simulink model "Katex_FullCar_R2017b_V03"  (R2026a)
settings: Solver=ode1  StopTime=1000  FixedStep=Ts  EnableMultiTasking=on
PostLoadFcn:
  | , if any(exist('dsrtsu_mdlpostloadfcn', 'file') == [2, 3, 6]), try dsrtsu_mdlpostloadfcn('Execute', bdroot); catch fprintf('Error in PostLoadFcn (dsrtsu_mdlpostloadfcn) for model "%s":\n %s\n', bdroot, lasterr); end, end,
  | , if any(exist('dsrtsu_mdlpostloadfcn', 'file') ~= 0), dsrtsu_mdlpostloadfcn('Execute', bdroot); end,
InitFcn:
  | , if any(exist('rtifpga_mdlclblib', 'file') ~= 0), rtifpga_mdlclblib('Init', bdroot); end,
  | 
  | 
  | init
undefined symbols (not defined in the file): locklim_sus, roundN, Ts
libraries: sl_discontinuities x29, simulink_extras x26, simulink x22, mjLib x1
(part 5 of 10)

== system Katex_FullCar_R2017b_V03/MuJoCo Interface/FR_Motor_Control/Str_Driver/Velocity Mode ==
  In1 : Inport
  Action Port : ActionPort  ActionPortLabel=elseif(u1 == 1)
  Constant : Constant  Value=0
  Terminator : Terminator
  Out1 : Outport  VectorParamsAs1DForOutWhenUnconnected=off
  wires:
  In1/1 -> Terminator/1
  Constant/1 -> Out1/1

== system Katex_FullCar_R2017b_V03/MuJoCo Interface/FR_Motor_Control/Sus_Driver/Position Mode ==
  In1 : Inport
  In2 : Inport  Port=2
  In3 : Inport  Port=3
  In4 : Inport  Port=4
  velocity_rad_s : Inport  Port=5
  Action Port : ActionPort  ActionPortLabel=if(u1 == 0)
  Bus Selector : BusSelector  OutputSignals=FRsus_angref_deg
  Degrees to Radians : simulink_extras/Transformations/Degrees to Radians
  FR_sus_position_motor_driver : Subsystem
  Out1 : Outport  VectorParamsAs1DForOutWhenUnconnected=off
  wires:
  velocity_rad_s/1 -> FR_sus_position_motor_driver/5(velocity_rad_s)
  In4/1 -> FR_sus_position_motor_driver/4(In4)
  In3/1 -> FR_sus_position_motor_driver/3(In3)
  In2/1 -> FR_sus_position_motor_driver/2(In2)
  Bus Selector/1 -> Degrees to Radians/1  "<FRsus_angref_deg>"
  In1/1 -> Bus Selector/1
  FR_sus_position_motor_driver/1(Out1) -> Out1/1
  Degrees to Radians/1 -> FR_sus_position_motor_driver/1(In1)

== system Katex_FullCar_R2017b_V03/MuJoCo Interface/FR_Motor_Control/Sus_Driver/Torque Mode ==
  In1 : Inport
  Action Port : ActionPort  ActionPortLabel=elseif(u1 == 2)
  Bus Selector1 : BusSelector  OutputSignals=FR_tqctrl.FRsus_tqref_pct
  controlgain : Outport  VectorParamsAs1DForOutWhenUnconnected=off
  wires:
  In1/1 -> Bus Selector1/1
  Bus Selector1/1 -> controlgain/1  "<FRsus_tqref_pct>"

== system Katex_FullCar_R2017b_V03/MuJoCo Interface/FR_Motor_Control/Sus_Driver/Velocity Mode ==
  In1 : Inport
  Action Port : ActionPort  ActionPortLabel=elseif(u1 == 1)
  Constant : Constant  Value=0
  Terminator : Terminator
  Out1 : Outport  VectorParamsAs1DForOutWhenUnconnected=off
  wires:
  In1/1 -> Terminator/1
  Constant/1 -> Out1/1

== system Katex_FullCar_R2017b_V03/MuJoCo Interface/RL_Motor_Control/Drv_Driver/Position Mode ==
  In1 : Inport
  Action Port : ActionPort  ActionPortLabel=if(u1 == 0)
  Constant : Constant  Value=0
  Terminator : Terminator
  Out1 : Outport  VectorParamsAs1DForOutWhenUnconnected=off
  wires:
  In1/1 -> Terminator/1
  Constant/1 -> Out1/1

== system Katex_FullCar_R2017b_V03/MuJoCo Interface/RL_Motor_Control/Drv_Driver/Torque Mode ==
  In1 : Inport
  Action Port : ActionPort  ActionPortLabel=elseif(u1 == 2)
  Bus Selector1 : BusSelector  OutputSignals=RL_tqctrl.RLdrv_tqref_pct
  controlgain : Outport  VectorParamsAs1DForOutWhenUnconnected=off
  wires:
  In1/1 -> Bus Selector1/1
  Bus Selector1/1 -> controlgain/1  "<RLdrv_tqref_pct>"

== system Katex_FullCar_R2017b_V03/MuJoCo Interface/RL_Motor_Control/Drv_Driver/Velocity Mode ==
  In1 : Inport
  In2 : Inport  Port=2
  In3 : Inport  Port=3
  In4 : Inport  Port=4
  In5 : Inport  Port=5
  Action Port : ActionPort  ActionPortLabel=elseif(u1 == 1)
  Bus Selector1 : BusSelector  OutputSignals=RLdrv_velref_mps
  RL_vel_velocity_motor_driver : Subsystem
  Subsystem13 : Subsystem
      mask Display: disp('Dri_ref(m/s)_2_motor(rad/s)');
  controlgain : Outport  VectorParamsAs1DForOutWhenUnconnected=off
  wires:
  In5/1 -> Subsystem13/2(In2)
  In4/1 -> RL_vel_velocity_motor_driver/4(In4)
  In3/1 -> RL_vel_velocity_motor_driver/3(In3)
  In2/1 -> RL_vel_velocity_motor_driver/2(In2)
  Subsystem13/1(Out1) -> RL_vel_velocity_motor_driver/1(In1)
  Bus Selector1/1 -> Subsystem13/1(In1)  "<RLdrv_velref_mps>"
  RL_vel_velocity_motor_driver/1(controlgain) -> controlgain/1
  In1/1 -> Bus Selector1/1

== system Katex_FullCar_R2017b_V03/MuJoCo Interface/RL_Motor_Control/Str_Driver/Position Mode ==
  In1 : Inport
  In2 : Inport  Port=2
  In3 : Inport  Port=3
  In4 : Inport  Port=4
  velocity_rad_s : Inport  Port=5
  Action Port : ActionPort  ActionPortLabel=if(u1 == 0)
  Bus Selector1 : BusSelector  OutputSignals=RLstr_angref_deg
  Degrees to Radians1 : simulink_extras/Transformations/Degrees to Radians
  RL_str_position_motor_driver : Subsystem
  Out1 : Outport  VectorParamsAs1DForOutWhenUnconnected=off
  wires:
  velocity_rad_s/1 -> RL_str_position_motor_driver/5(velocity_rad_s)
  In4/1 -> RL_str_position_motor_driver/4(In4)
  In3/1 -> RL_str_position_motor_driver/3(In3)
  In2/1 -> RL_str_position_motor_driver/2(In2)
  RL_str_position_motor_driver/1(Out1) -> Out1/1
  Bus Selector1/1 -> Degrees to Radians1/1  "<RLstr_angref_deg>"
  Degrees to Radians1/1 -> RL_str_position_motor_driver/1(In1)
  In1/1 -> Bus Selector1/1

== system Katex_FullCar_R2017b_V03/MuJoCo Interface/RL_Motor_Control/Str_Driver/Torque Mode ==
  In1 : Inport
  Action Port : ActionPort  ActionPortLabel=elseif(u1 == 2)
  Bus Selector1 : BusSelector  OutputSignals=RL_tqctrl.RLstr_tqref_pct
  controlgain : Outport  VectorParamsAs1DForOutWhenUnconnected=off
  wires:
  Bus Selector1/1 -> controlgain/1  "<RLstr_tqref_pct>"
  In1/1 -> Bus Selector1/1

== system Katex_FullCar_R2017b_V03/MuJoCo Interface/RL_Motor_Control/Str_Driver/Velocity Mode ==
  In1 : Inport
  Action Port : ActionPort  ActionPortLabel=elseif(u1 == 1)
  Constant : Constant  Value=0
  Terminator : Terminator
  Out1 : Outport  VectorParamsAs1DForOutWhenUnconnected=off
  wires:
  In1/1 -> Terminator/1
  Constant/1 -> Out1/1

== system Katex_FullCar_R2017b_V03/MuJoCo Interface/RL_Motor_Control/Sus_Driver/Position Mode ==
  In1 : Inport
  In2 : Inport  Port=2
  In3 : Inport  Port=3
  In4 : Inport  Port=4
  velocity_rad_s : Inport  Port=5
  Action Port : ActionPort  ActionPortLabel=if(u1 == 0)
  Bus Selector : BusSelector  OutputSignals=RLsus_angref_deg
  Degrees to Radians : simulink_extras/Transformations/Degrees to Radians
  RL_sus_position_motor_driver : Subsystem
  Out1 : Outport  VectorParamsAs1DForOutWhenUnconnected=off
  wires:
  velocity_rad_s/1 -> RL_sus_position_motor_driver/5(velocity_rad_s)
  In4/1 -> RL_sus_position_motor_driver/4(In4)
  In3/1 -> RL_sus_position_motor_driver/3(In3)
  In2/1 -> RL_sus_position_motor_driver/2(In2)
  Bus Selector/1 -> Degrees to Radians/1  "<RLsus_angref_deg>"
  In1/1 -> Bus Selector/1
  RL_sus_position_motor_driver/1(Out1) -> Out1/1
  Degrees to Radians/1 -> RL_sus_position_motor_driver/1(In1)

== system Katex_FullCar_R2017b_V03/MuJoCo Interface/RL_Motor_Control/Sus_Driver/Torque Mode ==
  In1 : Inport
  Action Port : ActionPort  ActionPortLabel=elseif(u1 == 2)
  Bus Selector1 : BusSelector  OutputSignals=RL_tqctrl.RLsus_tqref_pct
  controlgain : Outport  VectorParamsAs1DForOutWhenUnconnected=off
  wires:
  In1/1 -> Bus Selector1/1
  Bus Selector1/1 -> controlgain/1  "<RLsus_tqref_pct>"

== system Katex_FullCar_R2017b_V03/MuJoCo Interface/RL_Motor_Control/Sus_Driver/Velocity Mode ==
  In1 : Inport
  Action Port : ActionPort  ActionPortLabel=elseif(u1 == 1)
  Constant : Constant  Value=0
  Terminator : Terminator
  Out1 : Outport  VectorParamsAs1DForOutWhenUnconnected=off
  wires:
  In1/1 -> Terminator/1
  Constant/1 -> Out1/1

== system Katex_FullCar_R2017b_V03/MuJoCo Interface/RR_Motor_Control/Drv_Driver/Position Mode ==
  In1 : Inport
  Action Port : ActionPort  ActionPortLabel=if(u1 == 0)
  Constant : Constant  Value=0
  Terminator : Terminator
  Out1 : Outport  VectorParamsAs1DForOutWhenUnconnected=off
  wires:
  In1/1 -> Terminator/1
  Constant/1 -> Out1/1

== system Katex_FullCar_R2017b_V03/MuJoCo Interface/RR_Motor_Control/Drv_Driver/Torque Mode ==
  In1 : Inport
  Action Port : ActionPort  ActionPortLabel=elseif(u1 == 2)
  Bus Selector1 : BusSelector  OutputSignals=RR_tqctrl.RRdrv_tqref_pct
  controlgain : Outport  VectorParamsAs1DForOutWhenUnconnected=off
  wires:
  In1/1 -> Bus Selector1/1
  Bus Selector1/1 -> controlgain/1  "<RRdrv_tqref_pct>"

== system Katex_FullCar_R2017b_V03/MuJoCo Interface/RR_Motor_Control/Drv_Driver/Velocity Mode ==
  In1 : Inport
  In2 : Inport  Port=2
  In3 : Inport  Port=3
  In4 : Inport  Port=4
  In5 : Inport  Port=5
  Action Port : ActionPort  ActionPortLabel=elseif(u1 == 1)
  Bus Selector1 : BusSelector  OutputSignals=RRdrv_velref_mps
  RR_vel_velocity_motor_driver : Subsystem
  Subsystem13 : Subsystem
      mask Display: disp('Dri_ref(m/s)_2_motor(rad/s)');
  controlgain : Outport  VectorParamsAs1DForOutWhenUnconnected=off
  wires:
  In5/1 -> Subsystem13/2(In2)
  In4/1 -> RR_vel_velocity_motor_driver/4(In4)
  In3/1 -> RR_vel_velocity_motor_driver/3(In3)
  In2/1 -> RR_vel_velocity_motor_driver/2(In2)
  Subsystem13/1(Out1) -> RR_vel_velocity_motor_driver/1(In1)
  Bus Selector1/1 -> Subsystem13/1(In1)  "<RRdrv_velref_mps>"
  RR_vel_velocity_motor_driver/1(controlgain) -> controlgain/1
  In1/1 -> Bus Selector1/1

== system Katex_FullCar_R2017b_V03/MuJoCo Interface/RR_Motor_Control/Str_Driver/Position Mode ==
  In1 : Inport
  In2 : Inport  Port=2
  In3 : Inport  Port=3
  In4 : Inport  Port=4
  velocity_rad_s : Inport  Port=5
  Action Port : ActionPort  ActionPortLabel=if(u1 == 0)
  Bus Selector1 : BusSelector  OutputSignals=RRstr_angref_deg
  Degrees to Radians1 : simulink_extras/Transformations/Degrees to Radians
  RR_str_position_motor_driver : Subsystem
  Out1 : Outport  VectorParamsAs1DForOutWhenUnconnected=off
  wires:
  velocity_rad_s/1 -> RR_str_position_motor_driver/5(velocity_rad_s)
  In4/1 -> RR_str_position_motor_driver/4(In4)
  In3/1 -> RR_str_position_motor_driver/3(In3)
  In2/1 -> RR_str_position_motor_driver/2(In2)
  RR_str_position_motor_driver/1(Out1) -> Out1/1
  Bus Selector1/1 -> Degrees to Radians1/1  "<RRstr_angref_deg>"
  Degrees to Radians1/1 -> RR_str_position_motor_driver/1(In1)
  In1/1 -> Bus Selector1/1

== system Katex_FullCar_R2017b_V03/MuJoCo Interface/RR_Motor_Control/Str_Driver/Torque Mode ==
  In1 : Inport
  Action Port : ActionPort  ActionPortLabel=elseif(u1 == 2)
  Bus Selector1 : BusSelector  OutputSignals=RR_tqctrl.RRstr_tqref_pct
  controlgain : Outport  VectorParamsAs1DForOutWhenUnconnected=off
  wires:
  Bus Selector1/1 -> controlgain/1  "<RRstr_tqref_pct>"
  In1/1 -> Bus Selector1/1

== system Katex_FullCar_R2017b_V03/MuJoCo Interface/RR_Motor_Control/Str_Driver/Velocity Mode ==
  In1 : Inport
  Action Port : ActionPort  ActionPortLabel=elseif(u1 == 1)
  Constant : Constant  Value=0
  Terminator : Terminator
  Out1 : Outport  VectorParamsAs1DForOutWhenUnconnected=off
  wires:
  In1/1 -> Terminator/1
  Constant/1 -> Out1/1

== system Katex_FullCar_R2017b_V03/MuJoCo Interface/RR_Motor_Control/Sus_Driver/Position Mode ==
  In1 : Inport
  In2 : Inport  Port=2
  In3 : Inport  Port=3
  In4 : Inport  Port=4
  velocity_rad_s : Inport  Port=5
  Action Port : ActionPort  ActionPortLabel=if(u1 == 0)
  Bus Selector : BusSelector  OutputSignals=RRsus_angref_deg
  Degrees to Radians : simulink_extras/Transformations/Degrees to Radians
  RR_sus_position_motor_driver : Subsystem
  Out1 : Outport  VectorParamsAs1DForOutWhenUnconnected=off
  wires:
  velocity_rad_s/1 -> RR_sus_position_motor_driver/5(velocity_rad_s)
  In4/1 -> RR_sus_position_motor_driver/4(In4)
  In3/1 -> RR_sus_position_motor_driver/3(In3)
  In2/1 -> RR_sus_position_motor_driver/2(In2)
  Bus Selector/1 -> Degrees to Radians/1  "<RRsus_angref_deg>"
  In1/1 -> Bus Selector/1
  RR_sus_position_motor_driver/1(Out1) -> Out1/1
  Degrees to Radians/1 -> RR_sus_position_motor_driver/1(In1)

== system Katex_FullCar_R2017b_V03/MuJoCo Interface/RR_Motor_Control/Sus_Driver/Torque Mode ==
  In1 : Inport
  Action Port : ActionPort  ActionPortLabel=elseif(u1 == 2)
  Bus Selector1 : BusSelector  OutputSignals=RR_tqctrl.RRsus_tqref_pct
  controlgain : Outport  VectorParamsAs1DForOutWhenUnconnected=off
  wires:
  In1/1 -> Bus Selector1/1
  Bus Selector1/1 -> controlgain/1  "<RRsus_tqref_pct>"

== system Katex_FullCar_R2017b_V03/MuJoCo Interface/RR_Motor_Control/Sus_Driver/Velocity Mode ==
  In1 : Inport
  Action Port : ActionPort  ActionPortLabel=elseif(u1 == 1)
  Constant : Constant  Value=0
  Terminator : Terminator
  Out1 : Outport  VectorParamsAs1DForOutWhenUnconnected=off
  wires:
  In1/1 -> Terminator/1
  Constant/1 -> Out1/1

== system Katex_FullCar_R2017b_V03/DGIST/_High_Level_Ctrl/Chassis_FB_ctrl/Slip contro FLl/Subsystem ==
  Dri_ref[rad/s] : Inport
  Dri_meas[m/s] : Inport  Port=2
  Kgain : Inport  Port=3
  Slip Limit : Inport  Port=4
  radius : Inport  Port=5
  Add : Sum  Inputs=+-
  Constant : Constant  Value=0
  Gain : Gain  Gain=-1
  Max : MinMax  Function=max  Inputs=2
  Min : MinMax  Inputs=2
  "P controller " : Subsystem
  Product : Product
  Product1 : Product
  Product2 : Product
  Saturation Dynamic : sl_discontinuities/Saturation Dynamic  OutMin=[]  OutMax=[]  OutDataTypeStr=Inherit: Same as second input  OutDataType=fixdt(1, 16)  OutScaling=2^-10  DoSatur=off
  Slip_2_omega_block : Subsystem
  Subsystem1 : Subsystem
  re_ref : Scope  NumInputPorts=2
      settings: DataLoggingVariableName=ScopeData3
  ref_meas : Scope  NumInputPorts=2
      settings: DataLoggingVariableName=ScopeData2
  slip ratio : Product  Inputs=*/
  slipratio_satslipratio : Scope  NumInputPorts=2
  omega* : Outport  VectorParamsAs1DForOutWhenUnconnected=off
  wires:
  Dri_meas[m/s]/1 -> ref_meas/2, Slip_2_omega_block/3(Dri_meas[m/s]), Add/2  "Dri_meas[m/s]"
  Kgain/1 -> "P controller "/2(In2)  "Kgain"
  Add/1 -> slip ratio/1, "P controller "/1(In1)  "error[m/s]"
  Slip Limit/1 -> Gain/1, Saturation Dynamic/1  "Slip Limit"
  Gain/1 -> Saturation Dynamic/3
  Saturation Dynamic/1 -> Max/1, slipratio_satslipratio/2, Min/2  "sat slip ratio"
  radius/1 -> Product1/2, Slip_2_omega_block/4(radius)  "radius"
  slip ratio/1 -> slipratio_satslipratio/1  "slip ratio"
  Dri_ref[rad/s]/1 -> [initial_ref], Product1/1  "Dri_ref[rad/s]"
  Product1/1 -> ref_meas/1, Product/2, re_ref/1, slip ratio/2, Add/1  "ref[m/s]"
  Product/1 -> re_ref/2  "re_ref[m/s]"
  Constant/1 -> Min/1, Max/2
  Max/1 -> Slip_2_omega_block/1("lambda+ ")
  Min/1 -> Slip_2_omega_block/2(lambda-)
  Slip_2_omega_block/1(omega*[rad/s]) -> Product/1, omega*/1
  Subsystem1/1(sign) -> Product2/2
  [initial_ref] -> Subsystem1/1(In1)
  "P controller "/1(Out1) -> Product2/1
  Product2/1 -> Saturation Dynamic/2

== system Katex_FullCar_R2017b_V03/DGIST/_High_Level_Ctrl/Chassis_FB_ctrl/Slip control FR/Subsystem ==
  Dri_ref[rad/s] : Inport
  Dri_meas[m/s] : Inport  Port=2
  Kgain : Inport  Port=3
  Slip Limit : Inport  Port=4
  radius : Inport  Port=5
  Add : Sum  Inputs=+-
  Constant : Constant  Value=0
  Gain : Gain  Gain=-1
  Max : MinMax  Function=max  Inputs=2
  Min : MinMax  Inputs=2
  "P controller " : Subsystem
  Product : Product
  Product1 : Product
  Product2 : Product
  Saturation Dynamic : sl_discontinuities/Saturation Dynamic  OutMin=[]  OutMax=[]  OutDataTypeStr=Inherit: Same as second input  OutDataType=fixdt(1, 16)  OutScaling=2^-10  DoSatur=off
  Slip_2_omega_block : Subsystem
  Subsystem1 : Subsystem
  re_ref : Scope  NumInputPorts=2
      settings: DataLoggingVariableName=ScopeData3
  ref_meas : Scope  NumInputPorts=2
      settings: DataLoggingVariableName=ScopeData2
  slip ratio : Product  Inputs=*/
  slipratio_satslipratio : Scope  NumInputPorts=2
  omega* : Outport  VectorParamsAs1DForOutWhenUnconnected=off
  wires:
  Product2/1 -> Saturation Dynamic/2
  "P controller "/1(Out1) -> Product2/1
  [initial_ref] -> Subsystem1/1(In1)
  Subsystem1/1(sign) -> Product2/2
  Slip_2_omega_block/1(omega*[rad/s]) -> omega*/1, Product/1
  Min/1 -> Slip_2_omega_block/2(lambda-)
  Max/1 -> Slip_2_omega_block/1("lambda+ ")
  Constant/1 -> Max/2, Min/1
  Product/1 -> re_ref/2  "re_ref[m/s]"
  Product1/1 -> Add/1, slip ratio/2, re_ref/1, Product/2, ref_meas/1  "ref[m/s]"
  Dri_ref[rad/s]/1 -> Product1/1, [initial_ref]  "Dri_ref[rad/s]"
  slip ratio/1 -> slipratio_satslipratio/1  "slip ratio"
  radius/1 -> Slip_2_omega_block/4(radius), Product1/2  "radius"
  Saturation Dynamic/1 -> Min/2, slipratio_satslipratio/2, Max/1  "sat slip ratio"
  Gain/1 -> Saturation Dynamic/3
  Slip Limit/1 -> Saturation Dynamic/1, Gain/1  "Slip Limit"
  Add/1 -> "P controller "/1(In1), slip ratio/1  "error[m/s]"
  Kgain/1 -> "P controller "/2(In2)  "Kgain"
  Dri_meas[m/s]/1 -> Add/2, Slip_2_omega_block/3(Dri_meas[m/s]), ref_meas/2  "Dri_meas[m/s]"

== system Katex_FullCar_R2017b_V03/DGIST/_High_Level_Ctrl/Chassis_FB_ctrl/Subsystem3/If Action Subsystem ==
  In1 : Inport
  Action Port : ActionPort  ActionPortLabel=if(u1 >= 0)
  Out1 : Outport  VectorParamsAs1DForOutWhenUnconnected=off
  wires:
  In1/1 -> Out1/1

== system Katex_FullCar_R2017b_V03/DGIST/_High_Level_Ctrl/Chassis_FB_ctrl/Subsystem3/If Action Subsystem1 ==
  In1 : Inport
  Action Port : ActionPort  ActionPortLabel=elseif(u1<0)
  Out1 : Outport  VectorParamsAs1DForOutWhenUnconnected=off
  wires:
  In1/1 -> Out1/1

== system Katex_FullCar_R2017b_V03/DGIST/_Low_Level_Ctrl/Driving_Low_Level_Controller/FB Mode/Dri_Loadradps_2_mps ==
  note: Load rad/s
  note: Load m/s
  In1 : Inport
  Product7 : Product
  wheel_radius1 : Constant  Value=0.15
  Out1 : Outport
  wires:
  Product7/1 -> Out1/1
  In1/1 -> Product7/1
  wheel_radius1/1 -> Product7/2

== system Katex_FullCar_R2017b_V03/DGIST/_Low_Level_Ctrl/Driving_Low_Level_Controller/FB Mode/Dri_Loadradps_2_mps1 ==
  note: Load rad/s
  note: Load m/s
  In1 : Inport
  Product7 : Product
  wheel_radius1 : Constant  Value=0.15
  Out1 : Outport
  wires:
  Product7/1 -> Out1/1
  In1/1 -> Product7/1
  wheel_radius1/1 -> Product7/2

== system Katex_FullCar_R2017b_V03/DGIST/_Low_Level_Ctrl/Driving_Low_Level_Controller/Torque Mode/Driving Wheel Control ==
  note: DOB => 이전 Unsaturated Torque를 사용하는게 아니고
      | 이전 실제 Applied/Saturation Torque를 사용 필요?
      | (생각해봐야함)
  note: okay
  note: okay
  note: okay
  Ref : Inport
  Measure : Inport  Port=2
  Add : Sum  Inputs=++-
  Add1 : Sum  Inputs=+-
  Constant : Constant  Value=0
  DOB(omega) : Subsystem
  Feedforward(omega) : Subsystem
  Poleplacement(PI)1 : Subsystem
  Subsystem : Subsystem
  Target Torque : Outport
  tag scope: DriFR_ctrl_FF=global, DriFR_ctrl_PID=global, DriFR_ctrl_Total=global, DriFR_ctrl_dhat=global
  wires:
  Ref/1 -> Add1/1, Feedforward(omega)/1(command)  "Load rad/s"
  [dri_ff_cutoff] -> Feedforward(omega)/2(LFP cutoff)
  Subsystem/1(Target Torque) -> Target Torque/1
  Feedforward(omega)/1(FF) -> [DriFR_ctrl_FF], Add/1
  Poleplacement(PI)1/1(feedback gain) -> [DriFR_ctrl_PID], Add/2
  [Sensor_wheel_angvel] -> DOB(omega)/2(Y_out(w))
  DOB(omega)/1(Dist_hat) -> [DriFR_ctrl_dhat], Add/3
  Add/1 -> DOB(omega)/1(U_in*(Tm)), [DriFR_ctrl_Total], Subsystem/1(N*m)
  [dri_ff_onoff] -> Feedforward(omega)/3(ControlOnOff)
  [dri_dob_onoff] -> DOB(omega)/4(ControlOnOff)
  [dri_dob_cutoff] -> DOB(omega)/3(CutoffFreq_Q)
  [dri_pid_zeta] -> Poleplacement(PI)1/3(zeta)
  Measure/1 -> Add1/2  "Load rad/s"
  Add1/1 -> Poleplacement(PI)1/1(error)
  [dri_pid_cutoff] -> Poleplacement(PI)1/2(BW)
  [dri_pid_onoff] -> Poleplacement(PI)1/4(ConstrolOnOff)
  Constant/1 -> Poleplacement(PI)1/5(ControlInputError)

== system Katex_FullCar_R2017b_V03/DGIST/_Low_Level_Ctrl/Driving_Low_Level_Controller/Velocity Mode/Dri_Loadradps_2_mps ==
  note: Load rad/s
  note: Load m/s
  In1 : Inport
  Product7 : Product
  wheel_radius1 : Constant  Value=0.15
  Out1 : Outport
  wires:
  Product7/1 -> Out1/1
  In1/1 -> Product7/1
  wheel_radius1/1 -> Product7/2

== system Katex_FullCar_R2017b_V03/DGIST/_Low_Level_Ctrl/Driving_Low_Level_Controller/Velocity Mode/Dri_Loadradps_2_mps1 ==
  note: Load rad/s
  note: Load m/s
  In1 : Inport
  Product7 : Product
  wheel_radius1 : Constant  Value=0.15
  Out1 : Outport
  wires:
  Product7/1 -> Out1/1
  In1/1 -> Product7/1
  wheel_radius1/1 -> Product7/2

== system Katex_FullCar_R2017b_V03/DGIST/_Low_Level_Ctrl/Driving_Low_Level_Controller/Velocity Mode/Dri_Loadradps_2_mps2 ==
  note: Load rad/s
  note: Load m/s
  In1 : Inport
  Product7 : Product
  wheel_radius1 : Constant  Value=0.15
  Out1 : Outport
  wires:
  Product7/1 -> Out1/1
  In1/1 -> Product7/1
  wheel_radius1/1 -> Product7/2

== system Katex_FullCar_R2017b_V03/DGIST/_Low_Level_Ctrl/Driving_Low_Level_Controller/Velocity Mode/Dri_Loadradps_2_mps3 ==
  note: Load rad/s
  note: Load m/s
  In1 : Inport
  Product7 : Product
  wheel_radius1 : Constant  Value=0.15
  Out1 : Outport
  wires:
  Product7/1 -> Out1/1
  In1/1 -> Product7/1
  wheel_radius1/1 -> Product7/2

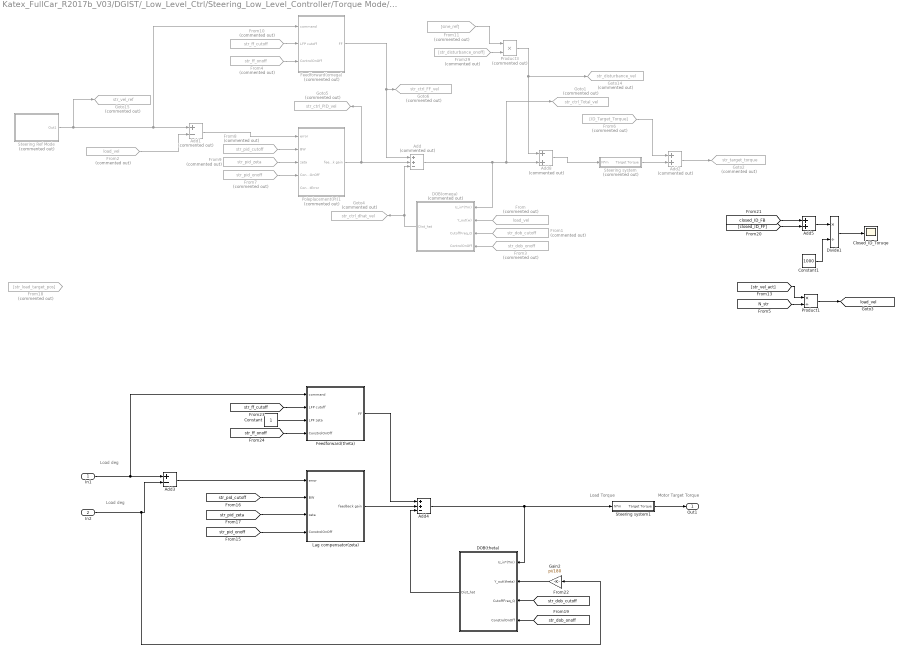
== system Katex_FullCar_R2017b_V03/DGIST/_Low_Level_Ctrl/Steering_Low_Level_Controller/Torque Mode/Steering Motor Control ==
  note: Load deg
  note: Load Torque
  note: Load deg
  note: Motor Target Torque
  In1 : Inport
  In2 : Inport  Port=2
  Add : Sum  Commented=on  Inputs=++-
  Add1 : Sum  Commented=on  Inputs=+-
  Add2 : Sum  Commented=on
  Add3 : Sum  Inputs=+-
  Add4 : Sum  Inputs=++-
  Add5 : Sum
  Add8 : Sum  Commented=on
  Closed_ID_Toruqe : Scope
  Constant : Constant
  Constant1 : Constant  Value=1000
  DOB(omega) : Subsystem  Commented=on
  DOB(theta) : Subsystem
  Divide1 : Product  Inputs=*/
  Feedforward(omega) : Subsystem  Commented=on
  Feedforward(theta) : Subsystem
  From : From  Commented=on  GotoTag=load_vel  TagVisibility=global
  From1 : From  Commented=on  GotoTag=str_dob_cutoff  TagVisibility=global
  From10 : From  Commented=on  GotoTag=str_ff_cutoff  TagVisibility=global
  From11 : From  Commented=on  GotoTag=sine_ref  TagVisibility=global
  From18 : From  Commented=on  GotoTag=str_load_target_pos  TagVisibility=global
  From2 : From  Commented=on  GotoTag=load_vel  TagVisibility=global
  From29 : From  Commented=on  GotoTag=str_disturbance_onoff  TagVisibility=global
  From3 : From  Commented=on  GotoTag=str_dob_onoff  TagVisibility=global
  From4 : From  Commented=on  GotoTag=str_ff_onoff  TagVisibility=global
  From6 : From  Commented=on  GotoTag=ID_Target_Torque  TagVisibility=global
  From7 : From  Commented=on  GotoTag=str_pid_onoff  TagVisibility=global
  From8 : From  Commented=on  GotoTag=str_pid_cutoff  TagVisibility=global
  From9 : From  Commented=on  GotoTag=str_pid_zeta  TagVisibility=global
  Gain2 : Gain  Gain=pi/180
  Goto1 : Goto  Commented=on  GotoTag=str_ctrl_Total_vel  TagVisibility=global
  Goto14 : Goto  Commented=on  GotoTag=str_disturbance_vel  TagVisibility=global
  Goto15 : Goto  Commented=on  GotoTag=str_vel_ref  TagVisibility=global
  Goto2 : Goto  Commented=on  GotoTag=str_target_torque  TagVisibility=global
  Goto4 : Goto  Commented=on  GotoTag=str_ctrl_dhat_vel  TagVisibility=global
  Goto5 : Goto  Commented=on  GotoTag=str_ctrl_PID_vel  TagVisibility=global
  Goto6 : Goto  Commented=on  GotoTag=str_ctrl_FF_vel  TagVisibility=global
  Lag compensator(zeta) : Subsystem
  Poleplacement(PI)1 : Subsystem  Commented=on
  Product1 : Product  Inputs=*/
  Product3 : Product  Commented=on  Inputs=**
  "Steering Ref Mode " : Subsystem  Commented=on
      mask Display: disp('Steering Ref Mode')
  Steering system : Subsystem  Commented=on
  Steering system1 : Subsystem
  Out1 : Outport
  tag scope: load_vel=global
  wires:
  [closed_ID_FF] -> Add5/2
  From8/1 -> Poleplacement(PI)1/2(BW)
  From7/1 -> Poleplacement(PI)1/4(ConstrolOnOff)
  [closed_ID_FB] -> Add5/1
  "Steering Ref Mode "/1(Out1) -> Goto15/1, Feedforward(omega)/1(command), Add1/1
  From6/1 -> Add2/1
  Steering system/1(Target Torque) -> Add2/2
  Add1/1 -> Poleplacement(PI)1/1(error)
  From9/1 -> Poleplacement(PI)1/3(zeta)
  Add2/1 -> Goto2/1
  [N_str] -> Product1/2
  Product1/1 -> [load_vel]
  [str_vel_act] -> Product1/1
  From2/1 -> Add1/2
  Constant1/1 -> Divide1/2
  Add5/1 -> Divide1/1
  Divide1/1 -> Closed_ID_Toruqe/1
  Poleplacement(PI)1/1(feedback gain) -> Add/2, Goto5/1
  Add/1 -> Goto1/1, Add8/2, DOB(omega)/1(U_in*(Tm))
  From/1 -> DOB(omega)/2(Y_out(w))
  From3/1 -> DOB(omega)/4(ControlOnOff)
  From1/1 -> DOB(omega)/3(CutoffFreq_Q)
  DOB(omega)/1(Dist_hat) -> Add/3, Goto4/1
  From10/1 -> Feedforward(omega)/2(LFP cutoff)
  From4/1 -> Feedforward(omega)/3(ControlOnOff)
  Feedforward(omega)/1(FF) -> Goto6/1, Add/1
  [str_dob_onoff] -> DOB(theta)/4(ConstrolOnOff)
  Add4/1 -> Steering system1/1(N*m), DOB(theta)/1(U_in*(Tm))
  [str_pid_zeta] -> Lag compensator(zeta)/3(zeta)
  [str_pid_cutoff] -> Lag compensator(zeta)/2(BW)
  [str_dob_cutoff] -> DOB(theta)/3(CutoffFreq_Q)
  Add3/1 -> Lag compensator(zeta)/1(error)
  [str_pid_onoff] -> Lag compensator(zeta)/4(ConstrolOnOff)
  Lag compensator(zeta)/1(feedback gain) -> Add4/2
  Constant/1 -> Feedforward(theta)/3(LPF zeta)
  [str_ff_cutoff] -> Feedforward(theta)/2(LFP cutoff)
  [str_ff_onoff] -> Feedforward(theta)/4(ConstrolOnOff)
  DOB(theta)/1(Dist_hat) -> Add4/3
  Feedforward(theta)/1(FF) -> Add4/1
  Steering system1/1(Target Torque) -> Out1/1
  In1/1 -> Feedforward(theta)/1(command), Add3/1
  In2/1 -> Gain2/1, Add3/2
  Gain2/1 -> DOB(theta)/2(Y_out(theta))
  From29/1 -> Product3/2
  From11/1 -> Product3/1
  Product3/1 -> Goto14/1, Add8/1
  Add8/1 -> Steering system/1(N*m)

== system Katex_FullCar_R2017b_V03/DGIST/_Low_Level_Ctrl/Steering_Low_Level_Controller/Torque Mode/Steering Motor Control1 ==
  note: Load deg
  note: Load Torque
  note: Load deg
  note: Motor Target Torque
  In1 : Inport
  In2 : Inport  Port=2
  Add3 : Sum  Inputs=+-
  Add4 : Sum  Inputs=++-
  Constant : Constant
  DOB(theta) : Subsystem
  Feedforward(theta) : Subsystem
  Gain2 : Gain  Gain=pi/180
  Lag compensator(zeta) : Subsystem
  Steering system1 : Subsystem
  Out1 : Outport
  wires:
  [str_dob_onoff] -> DOB(theta)/4(ConstrolOnOff)
  [str_pid_zeta] -> Lag compensator(zeta)/3(zeta)
  [str_pid_cutoff] -> Lag compensator(zeta)/2(BW)
  [str_dob_cutoff] -> DOB(theta)/3(CutoffFreq_Q)
  Add3/1 -> Lag compensator(zeta)/1(error)
  [str_pid_onoff] -> Lag compensator(zeta)/4(ConstrolOnOff)
  Lag compensator(zeta)/1(feedback gain) -> Add4/2
  Constant/1 -> Feedforward(theta)/3(LPF zeta)
  [str_ff_cutoff] -> Feedforward(theta)/2(LFP cutoff)
  [str_ff_onoff] -> Feedforward(theta)/4(ConstrolOnOff)
  DOB(theta)/1(Dist_hat) -> Add4/3
  Feedforward(theta)/1(FF) -> Add4/1
  Steering system1/1(Target Torque) -> Out1/1
  In1/1 -> Feedforward(theta)/1(command), Add3/1
  In2/1 -> Gain2/1, Add3/2
  Gain2/1 -> DOB(theta)/2(Y_out(theta))
  Add4/1 -> Steering system1/1(N*m), DOB(theta)/1(U_in*(Tm))

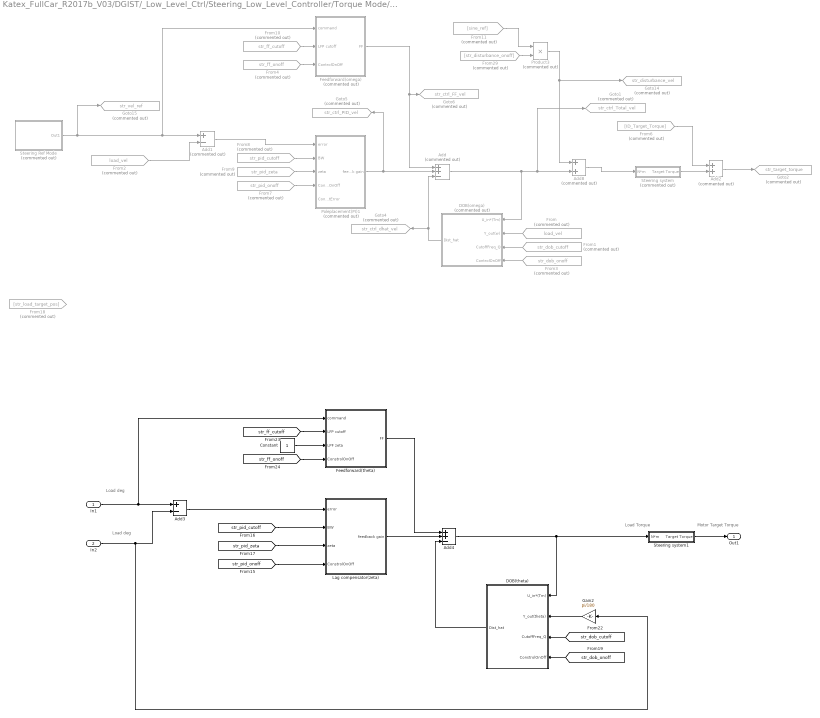
== system Katex_FullCar_R2017b_V03/DGIST/_Low_Level_Ctrl/Steering_Low_Level_Controller/Torque Mode/Steering Motor Control2 ==
  note: Load deg
  note: Load Torque
  note: Load deg
  note: Motor Target Torque
  In1 : Inport
  In2 : Inport  Port=2
  Add : Sum  Commented=on  Inputs=++-
  Add1 : Sum  Commented=on  Inputs=+-
  Add2 : Sum  Commented=on
  Add3 : Sum  Inputs=+-
  Add4 : Sum  Inputs=++-
  Add8 : Sum  Commented=on
  Constant : Constant
  DOB(omega) : Subsystem  Commented=on
  DOB(theta) : Subsystem
  Feedforward(omega) : Subsystem  Commented=on
  Feedforward(theta) : Subsystem
  From : From  Commented=on  GotoTag=load_vel  TagVisibility=global
  From1 : From  Commented=on  GotoTag=str_dob_cutoff  TagVisibility=global
  From10 : From  Commented=on  GotoTag=str_ff_cutoff  TagVisibility=global
  From11 : From  Commented=on  GotoTag=sine_ref  TagVisibility=global
  From18 : From  Commented=on  GotoTag=str_load_target_pos  TagVisibility=global
  From2 : From  Commented=on  GotoTag=load_vel  TagVisibility=global
  From29 : From  Commented=on  GotoTag=str_disturbance_onoff  TagVisibility=global
  From3 : From  Commented=on  GotoTag=str_dob_onoff  TagVisibility=global
  From4 : From  Commented=on  GotoTag=str_ff_onoff  TagVisibility=global
  From6 : From  Commented=on  GotoTag=ID_Target_Torque  TagVisibility=global
  From7 : From  Commented=on  GotoTag=str_pid_onoff  TagVisibility=global
  From8 : From  Commented=on  GotoTag=str_pid_cutoff  TagVisibility=global
  From9 : From  Commented=on  GotoTag=str_pid_zeta  TagVisibility=global
  Gain2 : Gain  Gain=pi/180
  Goto1 : Goto  Commented=on  GotoTag=str_ctrl_Total_vel  TagVisibility=global
  Goto14 : Goto  Commented=on  GotoTag=str_disturbance_vel  TagVisibility=global
  Goto15 : Goto  Commented=on  GotoTag=str_vel_ref  TagVisibility=global
  Goto2 : Goto  Commented=on  GotoTag=str_target_torque  TagVisibility=global
  Goto4 : Goto  Commented=on  GotoTag=str_ctrl_dhat_vel  TagVisibility=global
  Goto5 : Goto  Commented=on  GotoTag=str_ctrl_PID_vel  TagVisibility=global
  Goto6 : Goto  Commented=on  GotoTag=str_ctrl_FF_vel  TagVisibility=global
  Lag compensator(zeta) : Subsystem
  Poleplacement(PI)1 : Subsystem  Commented=on
  Product3 : Product  Commented=on  Inputs=**
  "Steering Ref Mode " : Subsystem  Commented=on
      mask Display: disp('Steering Ref Mode')
  Steering system : Subsystem  Commented=on
  Steering system1 : Subsystem
  Out1 : Outport
  wires:
  From8/1 -> Poleplacement(PI)1/2(BW)
  From7/1 -> Poleplacement(PI)1/4(ConstrolOnOff)
  "Steering Ref Mode "/1(Out1) -> Goto15/1, Feedforward(omega)/1(command), Add1/1
  From6/1 -> Add2/1
  Steering system/1(Target Torque) -> Add2/2
  Add1/1 -> Poleplacement(PI)1/1(error)
  From9/1 -> Poleplacement(PI)1/3(zeta)
  Add2/1 -> Goto2/1
  From2/1 -> Add1/2
  Poleplacement(PI)1/1(feedback gain) -> Add/2, Goto5/1
  Add/1 -> Goto1/1, Add8/2, DOB(omega)/1(U_in*(Tm))
  From/1 -> DOB(omega)/2(Y_out(w))
  From3/1 -> DOB(omega)/4(ControlOnOff)
  From1/1 -> DOB(omega)/3(CutoffFreq_Q)
  DOB(omega)/1(Dist_hat) -> Add/3, Goto4/1
  From10/1 -> Feedforward(omega)/2(LFP cutoff)
  From4/1 -> Feedforward(omega)/3(ControlOnOff)
  Feedforward(omega)/1(FF) -> Goto6/1, Add/1
  [str_dob_onoff] -> DOB(theta)/4(ConstrolOnOff)
  [str_pid_zeta] -> Lag compensator(zeta)/3(zeta)
  [str_pid_cutoff] -> Lag compensator(zeta)/2(BW)
  [str_dob_cutoff] -> DOB(theta)/3(CutoffFreq_Q)
  Add3/1 -> Lag compensator(zeta)/1(error)
  [str_pid_onoff] -> Lag compensator(zeta)/4(ConstrolOnOff)
  Lag compensator(zeta)/1(feedback gain) -> Add4/2
  Constant/1 -> Feedforward(theta)/3(LPF zeta)
  [str_ff_cutoff] -> Feedforward(theta)/2(LFP cutoff)
  [str_ff_onoff] -> Feedforward(theta)/4(ConstrolOnOff)
  DOB(theta)/1(Dist_hat) -> Add4/3
  Feedforward(theta)/1(FF) -> Add4/1
  Steering system1/1(Target Torque) -> Out1/1
  In1/1 -> Feedforward(theta)/1(command), Add3/1
  In2/1 -> Gain2/1, Add3/2
  Gain2/1 -> DOB(theta)/2(Y_out(theta))
  Add4/1 -> Steering system1/1(N*m), DOB(theta)/1(U_in*(Tm))
  From29/1 -> Product3/2
  From11/1 -> Product3/1
  Product3/1 -> Goto14/1, Add8/1
  Add8/1 -> Steering system/1(N*m)

== system Katex_FullCar_R2017b_V03/DGIST/_Low_Level_Ctrl/Steering_Low_Level_Controller/Torque Mode/Steering Motor Control3 ==
  note: Load deg
  note: Load Torque
  note: Load deg
  note: Motor Target Torque
  In1 : Inport
  In2 : Inport  Port=2
  Add3 : Sum  Inputs=+-
  Add4 : Sum  Inputs=++-
  Constant : Constant
  DOB(theta) : Subsystem
  Feedforward(theta) : Subsystem
  Gain2 : Gain  Gain=pi/180
  Lag compensator(zeta) : Subsystem
  Steering system1 : Subsystem
  Out1 : Outport
  tag scope: str_ctrl_PID_pos=global, str_ctrl_dhat_pos=global
  wires:
  [str_dob_onoff] -> DOB(theta)/4(ConstrolOnOff)
  [str_pid_zeta] -> Lag compensator(zeta)/3(zeta)
  [str_pid_cutoff] -> Lag compensator(zeta)/2(BW)
  [str_dob_cutoff] -> DOB(theta)/3(CutoffFreq_Q)
  Add3/1 -> Lag compensator(zeta)/1(error)
  [str_pid_onoff] -> Lag compensator(zeta)/4(ConstrolOnOff)
  Lag compensator(zeta)/1(feedback gain) -> [str_ctrl_PID_pos], Add4/2
  Constant/1 -> Feedforward(theta)/3(LPF zeta)
  [str_ff_cutoff] -> Feedforward(theta)/2(LFP cutoff)
  [str_ff_onoff] -> Feedforward(theta)/4(ConstrolOnOff)
  DOB(theta)/1(Dist_hat) -> [str_ctrl_dhat_pos], Add4/3
  Feedforward(theta)/1(FF) -> Add4/1
  Steering system1/1(Target Torque) -> Out1/1
  In1/1 -> Feedforward(theta)/1(command), Add3/1
  In2/1 -> Gain2/1, Add3/2
  Gain2/1 -> DOB(theta)/2(Y_out(theta))
  Add4/1 -> Steering system1/1(N*m), DOB(theta)/1(U_in*(Tm))

== system Katex_FullCar_R2017b_V03/DGIST/_Low_Level_Ctrl/Suspension_Low_Level_Controller/Torque Mode/Subsystem ==
  Add : Sum
  Add3 : Sum  Inputs=+-
  Add4 : Sum  Inputs=++-
  Add6 : Sum  Inputs=+++
  Add7 : Sum
  Constant : Constant
  DOB(theta) : Subsystem
  Feedforward(theta) : Subsystem
  Gain : Gain  Gain=pi/180
  Gain1 : Gain  Gain=pi/180
  Gain2 : Gain  Gain=pi/180
  Lag compensator(zeta) : Subsystem
  Product : Product
  Product2 : Product  Inputs=**
  Sus Ref Mode : Subsystem
      mask Display: disp('SusRef Mode')
  Suspension system1 : Subsystem
  "arm_length " : Gain  Gain=0.15
  g_force : Gain  Gain=9.81
  tag scope: sus_ctrl_FF_pos=global, sus_ctrl_PID_pos=global, sus_ctrl_Total_pos=global, sus_ctrl_dhat_pos=global, sus_pos_ref=global, sus_target_torque=global
  wires:
  [sus_disturbance_onoff] -> Product2/2
  [sus_pid_onoff] -> Lag compensator(zeta)/4(ConstrolOnOff)
  Gain/1 -> Feedforward(theta)/1(command), Add3/1
  Sus Ref Mode/1(Out1) -> [sus_pos_ref], Gain/1
  [sus_pid_zeta] -> Lag compensator(zeta)/3(zeta)
  Product2/1 -> Add7/1
  Suspension system1/1(Target Torque) -> Add6/2
  Lag compensator(zeta)/1(feedback gain) -> [sus_ctrl_PID_pos], Add4/2
  [sus_dob_cutoff] -> DOB(theta)/3(CutoffFreq_Q)
  Add3/1 -> Lag compensator(zeta)/1(error)
  DOB(theta)/1(Dist_hat) -> [sus_ctrl_dhat_pos], Add4/3
  Feedforward(theta)/1(FF) -> [sus_ctrl_FF_pos], Add4/1
  [sine_ref] -> Product2/1
  [ID_Target_Torque] -> Add6/1
  [sus_load_pos_act] -> Gain2/1
  [sus_ff_onoff] -> Feedforward(theta)/4(ConstrolOnOff)
  Gain1/1 -> Add3/2
  Constant/1 -> Feedforward(theta)/3(LPF zeta)
  [sus_dob_onoff] -> DOB(theta)/4(ConstrolOnOff)
  Add6/1 -> [sus_target_torque]
  Gain2/1 -> DOB(theta)/2(Y_out(theta))
  Add4/1 -> [sus_ctrl_Total_pos], Add7/2, DOB(theta)/1(U_in*(Tm))
  [sus_pid_cutoff] -> Lag compensator(zeta)/2(BW)
  [sus_ff_cutoff] -> Feedforward(theta)/2(LFP cutoff)
  [sus_load_pos_act] -> Gain1/1
  "arm_length "/1 -> Product/1  "Nm"
  g_force/1 -> "arm_length "/1  "N"
  [gravity_mass] -> g_force/1  "kg"
  [gravity_CP_OnOff] -> Product/2
  Add/1 -> Suspension system1/1(N*m)
  Add7/1 -> Add/1
  Product/1 -> Add/2

== system Katex_FullCar_R2017b_V03/DGIST/_Low_Level_Ctrl/Suspension_Low_Level_Controller/Velocity Mode/Sus_LoadVel_2_MotorRPM ==
  note: RPM
  note: Motor rad/s
  note: Load rad/s
  In1 : Inport
  Constant2 : Constant  Value=60/(2*pi)
  Data Type Conversion1 : DataTypeConversion  SaturateOnIntegerOverflow=off  RndMeth=Floor
  Gain : Gain  Gain=-1
  LPF2 : Subsystem
  Product3 : Product
  Product4 : Product
  Rate Limiter Dynamic : sl_discontinuities/Rate Limiter Dynamic
  Saturation1 : Saturate  UpperLimit=70  LowerLimit=-70
  Out1 : Outport
  wires:
  Product3/1 -> Product4/1
  Product4/1 -> Data Type Conversion1/1
  [sus_vel_ref_cutoff] -> LPF2/2(fc)
  Gain/1 -> Rate Limiter Dynamic/3
  Constant2/1 -> Product4/2
  [sus_vel_ref_ratelimit] -> Gain/1, Rate Limiter Dynamic/1
  LPF2/1(Out) -> Product3/1
  [N_sus] -> Product3/2
  Saturation1/1 -> Rate Limiter Dynamic/2
  Rate Limiter Dynamic/1 -> LPF2/1(In)
  In1/1 -> Saturation1/1
  Data Type Conversion1/1 -> Out1/1

== system Katex_FullCar_R2017b_V03/DGIST/_Low_Level_Ctrl/Suspension_Low_Level_Controller/Velocity Mode/Sus_LoadVel_2_MotorRPM1 ==
  note: RPM
  note: Motor rad/s
  note: Load rad/s
  In1 : Inport
  Constant2 : Constant  Value=60/(2*pi)
  Data Type Conversion1 : DataTypeConversion  SaturateOnIntegerOverflow=off  RndMeth=Floor
  Gain : Gain  Gain=-1
  LPF2 : Subsystem
  Product3 : Product
  Product4 : Product
  Rate Limiter Dynamic : sl_discontinuities/Rate Limiter Dynamic
  Saturation1 : Saturate  UpperLimit=70  LowerLimit=-70
  Out1 : Outport
  wires:
  Product3/1 -> Product4/1
  Product4/1 -> Data Type Conversion1/1
  [sus_pos_ref_cutoff] -> LPF2/2(fc)
  Gain/1 -> Rate Limiter Dynamic/3
  Constant2/1 -> Product4/2
  [sus_pos_ref_ratelimit] -> Gain/1, Rate Limiter Dynamic/1
  LPF2/1(Out) -> Product3/1
  [N_sus] -> Product3/2
  Saturation1/1 -> Rate Limiter Dynamic/2
  Rate Limiter Dynamic/1 -> LPF2/1(In)
  In1/1 -> Saturation1/1
  Data Type Conversion1/1 -> Out1/1

== system Katex_FullCar_R2017b_V03/DGIST/_Low_Level_Ctrl/Suspension_Low_Level_Controller/Velocity Mode/Sus_LoadVel_2_MotorRPM2 ==
  note: RPM
  note: Motor rad/s
  note: Load rad/s
  In1 : Inport
  Constant2 : Constant  Value=60/(2*pi)
  Data Type Conversion1 : DataTypeConversion  SaturateOnIntegerOverflow=off  RndMeth=Floor
  Gain : Gain  Gain=-1
  LPF2 : Subsystem
  Product3 : Product
  Product4 : Product
  Rate Limiter Dynamic : sl_discontinuities/Rate Limiter Dynamic
  Saturation1 : Saturate  UpperLimit=70  LowerLimit=-70
  Out1 : Outport
  wires:
  Product3/1 -> Product4/1
  Product4/1 -> Data Type Conversion1/1
  [sus_pos_ref_cutoff] -> LPF2/2(fc)
  Gain/1 -> Rate Limiter Dynamic/3
  Constant2/1 -> Product4/2
  [sus_pos_ref_ratelimit] -> Gain/1, Rate Limiter Dynamic/1
  LPF2/1(Out) -> Product3/1
  [N_sus] -> Product3/2
  Saturation1/1 -> Rate Limiter Dynamic/2
  Rate Limiter Dynamic/1 -> LPF2/1(In)
  In1/1 -> Saturation1/1
  Data Type Conversion1/1 -> Out1/1

== system Katex_FullCar_R2017b_V03/DGIST/_Low_Level_Ctrl/Suspension_Low_Level_Controller/Velocity Mode/Sus_LoadVel_2_MotorRPM3 ==
  note: RPM
  note: Motor rad/s
  note: Load rad/s
  In1 : Inport
  Constant2 : Constant  Value=60/(2*pi)
  Data Type Conversion1 : DataTypeConversion  SaturateOnIntegerOverflow=off  RndMeth=Floor
  Gain : Gain  Gain=-1
  LPF2 : Subsystem
  Product3 : Product
  Product4 : Product
  Rate Limiter Dynamic : sl_discontinuities/Rate Limiter Dynamic
  Saturation1 : Saturate  UpperLimit=70  LowerLimit=-70
  Out1 : Outport
  wires:
  Product3/1 -> Product4/1
  Product4/1 -> Data Type Conversion1/1
  [sus_pos_ref_cutoff] -> LPF2/2(fc)
  Gain/1 -> Rate Limiter Dynamic/3
  Constant2/1 -> Product4/2
  [sus_pos_ref_ratelimit] -> Gain/1, Rate Limiter Dynamic/1
  LPF2/1(Out) -> Product3/1
  [N_sus] -> Product3/2
  Saturation1/1 -> Rate Limiter Dynamic/2
  Rate Limiter Dynamic/1 -> LPF2/1(In)
  In1/1 -> Saturation1/1
  Data Type Conversion1/1 -> Out1/1

== system Katex_FullCar_R2017b_V03/MuJoCo Interface/FL_Motor_Control/Drv_Driver/Velocity Mode/FL_vel_velocity_motor_driver ==
  In1 : Inport
  In2 : Inport  Port=2
  In3 : Inport  Port=3
  In4 : Inport  Port=4
  Add : Sum  Inputs=-+
  Saturation : Saturate  UpperLimit=100  LowerLimit=-100
  Sum1 : Sum  Inputs=|+-
  poleplacement(PI)1 : Subsystem
  controlgain : Outport
  wires:
  Add/1 -> poleplacement(PI)1/4(anti_windup)
  Saturation/1 -> Add/1, controlgain/1
  In2/1 -> poleplacement(PI)1/2(zeta)
  In4/1 -> Sum1/2
  In1/1 -> Sum1/1
  In3/1 -> poleplacement(PI)1/3(freq)
  Sum1/1 -> poleplacement(PI)1/1(error)
  poleplacement(PI)1/1(controlgain) -> Saturation/1, Add/2

== system Katex_FullCar_R2017b_V03/MuJoCo Interface/FL_Motor_Control/Drv_Driver/Velocity Mode/Subsystem13 ==
  In1 : Inport
  In2 : Inport  Port=2
  Product : Product  Inputs=*/
  Out1 : Outport
  wires:
  In2/1 -> Product/2
  Product/1 -> Out1/1  "Load (rad/s)"
  In1/1 -> Product/1  "m/s"

== system Katex_FullCar_R2017b_V03/MuJoCo Interface/FL_Motor_Control/Str_Driver/Position Mode/FL_str_position_motor_driver ==
  In1 : Inport
  In2 : Inport  Port=2
  In3 : Inport  Port=3
  In4 : Inport  Port=4
  velocity_rad_s : Inport  Port=5
  Sum1 : Sum  Inputs=|+-
  poleplacement(PD)+I : Subsystem
  Out1 : Outport
  wires:
  poleplacement(PD)+I/1(controlgain) -> Out1/1
  In2/1 -> poleplacement(PD)+I/2(zeta)
  Sum1/1 -> poleplacement(PD)+I/1(error)
  In3/1 -> poleplacement(PD)+I/3(freq)
  In1/1 -> Sum1/1
  In4/1 -> Sum1/2
  velocity_rad_s/1 -> poleplacement(PD)+I/4(velocity_rad_s)

== system Katex_FullCar_R2017b_V03/MuJoCo Interface/FL_Motor_Control/Sus_Driver/Position Mode/FL_sus_position_motor_driver ==
  In1 : Inport
  In2 : Inport  Port=2
  In3 : Inport  Port=3
  In4 : Inport  Port=4
  velocity_rad_s : Inport  Port=5
  Sum : Sum  Inputs=|+-
  poleplacement(PD)+I : Subsystem
  Out1 : Outport
  wires:
  In4/1 -> Sum/2
  Sum/1 -> poleplacement(PD)+I/1(error)
  poleplacement(PD)+I/1(controlgain) -> Out1/1
  In1/1 -> Sum/1
  In2/1 -> poleplacement(PD)+I/2(zeta)
  In3/1 -> poleplacement(PD)+I/3(freq)
  velocity_rad_s/1 -> poleplacement(PD)+I/4(velocity_rad_s)

== system Katex_FullCar_R2017b_V03/MuJoCo Interface/FR_Motor_Control/Drv_Driver/Velocity Mode/FR_vel_velocity_motor_driver ==
  In1 : Inport
  In2 : Inport  Port=2
  In3 : Inport  Port=3
  In4 : Inport  Port=4
  Add : Sum  Inputs=-+
  Saturation : Saturate  UpperLimit=100  LowerLimit=-100
  Sum1 : Sum  Inputs=|+-
  poleplacement(PI)1 : Subsystem
  controlgain : Outport
  wires:
  poleplacement(PI)1/1(controlgain) -> Add/2, Saturation/1
  Sum1/1 -> poleplacement(PI)1/1(error)
  In3/1 -> poleplacement(PI)1/3(freq)
  In1/1 -> Sum1/1
  In4/1 -> Sum1/2
  In2/1 -> poleplacement(PI)1/2(zeta)
  Saturation/1 -> controlgain/1, Add/1
  Add/1 -> poleplacement(PI)1/4(anti_windup)

== system Katex_FullCar_R2017b_V03/MuJoCo Interface/FR_Motor_Control/Drv_Driver/Velocity Mode/Subsystem13 ==
  In1 : Inport
  In2 : Inport  Port=2
  Product : Product  Inputs=*/
  Out1 : Outport
  wires:
  In1/1 -> Product/1  "m/s"
  Product/1 -> Out1/1  "Load (rad/s)"
  In2/1 -> Product/2

== system Katex_FullCar_R2017b_V03/MuJoCo Interface/FR_Motor_Control/Str_Driver/Position Mode/FR_str_position_motor_driver ==
  In1 : Inport
  In2 : Inport  Port=2
  In3 : Inport  Port=3
  In4 : Inport  Port=4
  velocity_rad_s : Inport  Port=5
  Sum1 : Sum  Inputs=|+-
  poleplacement(PD)+I : Subsystem
  Out1 : Outport
  wires:
  velocity_rad_s/1 -> poleplacement(PD)+I/4(velocity_rad_s)
  In4/1 -> Sum1/2
  In1/1 -> Sum1/1
  In3/1 -> poleplacement(PD)+I/3(freq)
  Sum1/1 -> poleplacement(PD)+I/1(error)
  In2/1 -> poleplacement(PD)+I/2(zeta)
  poleplacement(PD)+I/1(controlgain) -> Out1/1

== system Katex_FullCar_R2017b_V03/MuJoCo Interface/FR_Motor_Control/Sus_Driver/Position Mode/FR_sus_position_motor_driver ==
  In1 : Inport
  In2 : Inport  Port=2
  In3 : Inport  Port=3
  In4 : Inport  Port=4
  velocity_rad_s : Inport  Port=5
  Sum : Sum  Inputs=|+-
  poleplacement(PD)+I : Subsystem
  Out1 : Outport
  wires:
  velocity_rad_s/1 -> poleplacement(PD)+I/4(velocity_rad_s)
  In3/1 -> poleplacement(PD)+I/3(freq)
  In2/1 -> poleplacement(PD)+I/2(zeta)
  In1/1 -> Sum/1
  poleplacement(PD)+I/1(controlgain) -> Out1/1
  Sum/1 -> poleplacement(PD)+I/1(error)
  In4/1 -> Sum/2

== system Katex_FullCar_R2017b_V03/MuJoCo Interface/RL_Motor_Control/Drv_Driver/Velocity Mode/RL_vel_velocity_motor_driver ==
  In1 : Inport
  In2 : Inport  Port=2
  In3 : Inport  Port=3
  In4 : Inport  Port=4
  Add : Sum  Inputs=-+
  Saturation : Saturate  UpperLimit=100  LowerLimit=-100
  Sum1 : Sum  Inputs=|+-
  poleplacement(PI)1 : Subsystem
  controlgain : Outport
  wires:
  poleplacement(PI)1/1(controlgain) -> Add/2, Saturation/1
  Sum1/1 -> poleplacement(PI)1/1(error)
  In3/1 -> poleplacement(PI)1/3(freq)
  In1/1 -> Sum1/1
  In4/1 -> Sum1/2
  In2/1 -> poleplacement(PI)1/2(zeta)
  Saturation/1 -> controlgain/1, Add/1
  Add/1 -> poleplacement(PI)1/4(anti_windup)

== system Katex_FullCar_R2017b_V03/MuJoCo Interface/RL_Motor_Control/Drv_Driver/Velocity Mode/Subsystem13 ==
  In1 : Inport
  In2 : Inport  Port=2
  Product : Product  Inputs=*/
  Out1 : Outport
  wires:
  In1/1 -> Product/1  "m/s"
  Product/1 -> Out1/1  "Load (rad/s)"
  In2/1 -> Product/2

== system Katex_FullCar_R2017b_V03/MuJoCo Interface/RL_Motor_Control/Str_Driver/Position Mode/RL_str_position_motor_driver ==
  In1 : Inport
  In2 : Inport  Port=2
  In3 : Inport  Port=3
  In4 : Inport  Port=4
  velocity_rad_s : Inport  Port=5
  Sum1 : Sum  Inputs=|+-
  poleplacement(PD)+I : Subsystem
  Out1 : Outport
  wires:
  velocity_rad_s/1 -> poleplacement(PD)+I/4(velocity_rad_s)
  In4/1 -> Sum1/2
  In1/1 -> Sum1/1
  In3/1 -> poleplacement(PD)+I/3(freq)
  Sum1/1 -> poleplacement(PD)+I/1(error)
  In2/1 -> poleplacement(PD)+I/2(zeta)
  poleplacement(PD)+I/1(controlgain) -> Out1/1

== system Katex_FullCar_R2017b_V03/MuJoCo Interface/RL_Motor_Control/Sus_Driver/Position Mode/RL_sus_position_motor_driver ==
  In1 : Inport
  In2 : Inport  Port=2
  In3 : Inport  Port=3
  In4 : Inport  Port=4
  velocity_rad_s : Inport  Port=5
  Sum : Sum  Inputs=|+-
  poleplacement(PD)+I : Subsystem
  Out1 : Outport
  wires:
  velocity_rad_s/1 -> poleplacement(PD)+I/4(velocity_rad_s)
  In3/1 -> poleplacement(PD)+I/3(freq)
  In2/1 -> poleplacement(PD)+I/2(zeta)
  In1/1 -> Sum/1
  poleplacement(PD)+I/1(controlgain) -> Out1/1
  Sum/1 -> poleplacement(PD)+I/1(error)
  In4/1 -> Sum/2

== system Katex_FullCar_R2017b_V03/MuJoCo Interface/RR_Motor_Control/Drv_Driver/Velocity Mode/RR_vel_velocity_motor_driver ==
  In1 : Inport
  In2 : Inport  Port=2
  In3 : Inport  Port=3
  In4 : Inport  Port=4
  Add : Sum  Inputs=-+
  Saturation : Saturate  UpperLimit=100  LowerLimit=-100
  Sum1 : Sum  Inputs=|+-
  poleplacement(PI)1 : Subsystem
  controlgain : Outport
  wires:
  poleplacement(PI)1/1(controlgain) -> Add/2, Saturation/1
  Sum1/1 -> poleplacement(PI)1/1(error)
  In3/1 -> poleplacement(PI)1/3(freq)
  In1/1 -> Sum1/1
  In4/1 -> Sum1/2
  In2/1 -> poleplacement(PI)1/2(zeta)
  Saturation/1 -> controlgain/1, Add/1
  Add/1 -> poleplacement(PI)1/4(anti_windup)

== system Katex_FullCar_R2017b_V03/MuJoCo Interface/RR_Motor_Control/Drv_Driver/Velocity Mode/Subsystem13 ==
  In1 : Inport
  In2 : Inport  Port=2
  Product : Product  Inputs=*/
  Out1 : Outport
  wires:
  In1/1 -> Product/1  "m/s"
  Product/1 -> Out1/1  "Load (rad/s)"
  In2/1 -> Product/2

== system Katex_FullCar_R2017b_V03/MuJoCo Interface/RR_Motor_Control/Str_Driver/Position Mode/RR_str_position_motor_driver ==
  In1 : Inport
  In2 : Inport  Port=2
  In3 : Inport  Port=3
  In4 : Inport  Port=4
  velocity_rad_s : Inport  Port=5
  Sum1 : Sum  Inputs=|+-
  poleplacement(PD)+I : Subsystem
  Out1 : Outport
  wires:
  velocity_rad_s/1 -> poleplacement(PD)+I/4(velocity_rad_s)
  In4/1 -> Sum1/2
  In1/1 -> Sum1/1
  In3/1 -> poleplacement(PD)+I/3(freq)
  Sum1/1 -> poleplacement(PD)+I/1(error)
  In2/1 -> poleplacement(PD)+I/2(zeta)
  poleplacement(PD)+I/1(controlgain) -> Out1/1

== system Katex_FullCar_R2017b_V03/MuJoCo Interface/RR_Motor_Control/Sus_Driver/Position Mode/RR_sus_position_motor_driver ==
  In1 : Inport
  In2 : Inport  Port=2
  In3 : Inport  Port=3
  In4 : Inport  Port=4
  velocity_rad_s : Inport  Port=5
  Sum : Sum  Inputs=|+-
  poleplacement(PD)+I : Subsystem
  Out1 : Outport
  wires:
  velocity_rad_s/1 -> poleplacement(PD)+I/4(velocity_rad_s)
  In3/1 -> poleplacement(PD)+I/3(freq)
  In2/1 -> poleplacement(PD)+I/2(zeta)
  In1/1 -> Sum/1
  poleplacement(PD)+I/1(controlgain) -> Out1/1
  Sum/1 -> poleplacement(PD)+I/1(error)
  In4/1 -> Sum/2

== system Katex_FullCar_R2017b_V03/DGIST/_High_Level_Ctrl/Chassis_FB_ctrl/Slip contro FLl/Subsystem/P controller  ==
  In1 : Inport
  In2 : Inport  Port=2
  Product : Product
  Out1 : Outport  VectorParamsAs1DForOutWhenUnconnected=off
  wires:
  In1/1 -> Product/1
  In2/1 -> Product/2
  Product/1 -> Out1/1

== system Katex_FullCar_R2017b_V03/DGIST/_High_Level_Ctrl/Chassis_FB_ctrl/Slip contro FLl/Subsystem/Slip_2_omega_block ==
  "lambda+ " : Inport
  lambda- : Inport  Port=2
  Dri_meas[m/s] : Inport  Port=3
  radius : Inport  Port=4
  Add : Sum
  Add1 : Sum  Inputs=+-
  Constant : Constant
  Product : Product  Inputs=*/
  Product1 : Product  Inputs=**/
  omega*[rad/s] : Outport  VectorParamsAs1DForOutWhenUnconnected=off
  wires:
  Product1/1 -> omega*[rad/s]/1
  radius/1 -> Product/2
  Dri_meas[m/s]/1 -> Product/1
  "lambda+ "/1 -> Add1/2
  Constant/1 -> Add/1, Add1/1
  lambda-/1 -> Add/2
  Product/1 -> Product1/2
  Add/1 -> Product1/1
  Add1/1 -> Product1/3

== system Katex_FullCar_R2017b_V03/DGIST/_High_Level_Ctrl/Chassis_FB_ctrl/Slip contro FLl/Subsystem/Subsystem1 ==
  In1 : Inport
  Constant2 : Constant
  Constant3 : Constant  Value=-1
  If : If  IfExpression=u1 >= 0  ElseIfExpressions=u1<0
  If Action Subsystem : Subsystem  TreatAsAtomicUnit=on
  If Action Subsystem1 : Subsystem  TreatAsAtomicUnit=on
  Merge : Merge
  sign : Outport  VectorParamsAs1DForOutWhenUnconnected=off
  wires:
  If/1 -> If Action Subsystem/Action
  If/2 -> If Action Subsystem1/Action
  Constant2/1 -> If Action Subsystem/1(In1)
  Merge/1 -> sign/1
  In1/1 -> If/1
  Constant3/1 -> If Action Subsystem1/1(In1)
  If Action Subsystem1/1(Out1) -> Merge/2
  If Action Subsystem/1(Out1) -> Merge/1

== system Katex_FullCar_R2017b_V03/DGIST/_High_Level_Ctrl/Chassis_FB_ctrl/Slip control FR/Subsystem/P controller  ==
  In1 : Inport
  In2 : Inport  Port=2
  Product : Product
  Out1 : Outport  VectorParamsAs1DForOutWhenUnconnected=off
  wires:
  Product/1 -> Out1/1
  In2/1 -> Product/2
  In1/1 -> Product/1

== system Katex_FullCar_R2017b_V03/DGIST/_High_Level_Ctrl/Chassis_FB_ctrl/Slip control FR/Subsystem/Slip_2_omega_block ==
  "lambda+ " : Inport
  lambda- : Inport  Port=2
  Dri_meas[m/s] : Inport  Port=3
  radius : Inport  Port=4
  Add : Sum
  Add1 : Sum  Inputs=+-
  Constant : Constant
  Product : Product  Inputs=*/
  Product1 : Product  Inputs=**/
  omega*[rad/s] : Outport  VectorParamsAs1DForOutWhenUnconnected=off
  wires:
  Add1/1 -> Product1/3
  Add/1 -> Product1/1
  Product/1 -> Product1/2
  lambda-/1 -> Add/2
  Constant/1 -> Add1/1, Add/1
  "lambda+ "/1 -> Add1/2
  Dri_meas[m/s]/1 -> Product/1
  radius/1 -> Product/2
  Product1/1 -> omega*[rad/s]/1
